simulink model "pendelbeo"  (R2012b)
settings: Solver=ode45  StartTime=0.0  StopTime=10.0  RelTol=1e-3
undefined symbols (not defined in the file): g, J_S0, l, m, M, p, x1, x2, x3, x4
libraries: commnoisgen2 x1
settings Model: Creator=Pendel  LastModifiedBy=Pendel

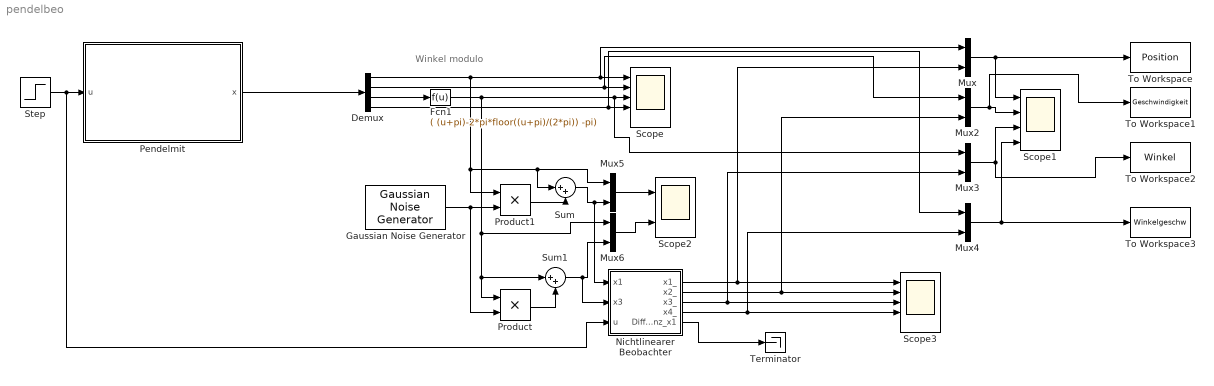
== system pendelbeo ==
  note: Winkel modulo
  Demux : Demux
  Fcn1 : Fcn  Expr=( (u+pi)-2*pi*floor((u+pi)/(2*pi)) -pi)
  Gaussian Noise Generator : commnoisgen2/Gaussian Noise Generator  m=0  d=0.0008  s=0  Ts=1e-3  frameBased=off  sampPerFrame=1  orient=off  outDataType=double
  Mux{,2..6} (6 alike) : Mux  Inputs=2
  Nichtlinearer Beobachter : Subsystem
  Pendelmit : Subsystem
  Product : Product  RndMeth=Zero
  Product1 : Product  RndMeth=Zero
  Scope : Scope  NumInputPorts=5
      settings: TimeRange=100  YMin=-0.5~-2~-5~-20~-200  YMax=1~1~5~40~200  SaveName=simulation_data  MaxDataPoints=500000
  Scope1 : Scope  NumInputPorts=4
      settings: TimeRange=3.23208722741433  YMin=-0.0035~-0.02~-0.0025~-0.0125  YMax=0.003~0.025~0.0025~0.015  SaveName=simulation_data2  MaxDataPoints=500000
  Scope2 : Scope  NumInputPorts=2
      settings: TimeRange=100  YMin=-0.5~-5  YMax=1~5  SaveName=simulation_data4  MaxDataPoints=500000
  Scope3 : Scope  NumInputPorts=5
      settings: TimeRange=25  YMin=-0.5~-2~-4~-200~-1  YMax=0.5~2~4~200~1  SaveName=simulation_data1  MaxDataPoints=500000
  Step : Step  SampleTime=0
  Sum : Sum  Inputs=|++
  Sum1 : Sum  Inputs=|++
  Terminator : Terminator
  To Workspace : ToWorkspace  VariableName=Position  SampleTime=-1  SaveFormat=Timeseries
  To Workspace1 : ToWorkspace  VariableName=Geschwindigkeit  SampleTime=-1  SaveFormat=Timeseries
  To Workspace2 : ToWorkspace  VariableName=Winkel  SampleTime=-1  SaveFormat=Timeseries
  To Workspace3 : ToWorkspace  VariableName=Winkelgeschw  SampleTime=-1  SaveFormat=Timeseries
  wires:
  Demux/1 -> Mux5/1, Sum/1, Product1/1, Mux/1, Scope/1
  Demux/4 -> Mux4/1, Scope/4
  Demux/2 -> Mux2/1, Scope/2
  Demux/3 -> Fcn1/1
  Fcn1/1 -> Mux6/1, Sum1/1, Product/1, Mux3/1, Scope/3
  Pendelmit/1(x) -> Demux/1
  Nichtlinearer Beobachter/1(x1_) -> Mux/2, Scope3/1
  Nichtlinearer Beobachter/2(x2_) -> Mux2/2, Scope3/2
  Nichtlinearer Beobachter/3(x3_) -> Mux3/2, Scope3/3
  Nichtlinearer Beobachter/4(x4_) -> Mux4/2, Scope3/4
  Mux3/1 -> Scope1/3, To Workspace2/1
  Mux/1 -> To Workspace/1, Scope1/1
  Mux4/1 -> To Workspace3/1, Scope1/4
  Mux5/1 -> Scope2/1
  Mux6/1 -> Scope2/2
  Gaussian Noise Generator/1 -> Product1/2, Product/2
  Sum/1 -> Nichtlinearer Beobachter/1(x1), Mux5/2
  Sum1/1 -> Nichtlinearer Beobachter/2(x3), Mux6/2
  Nichtlinearer Beobachter/5(Differenz_x1) -> Terminator/1
  Step/1 -> Nichtlinearer Beobachter/3(u), Pendelmit/1(u)
  Mux2/1 -> To Workspace1/1, Scope1/2
  Product1/1 -> Sum/2
  Product/1 -> Sum1/2

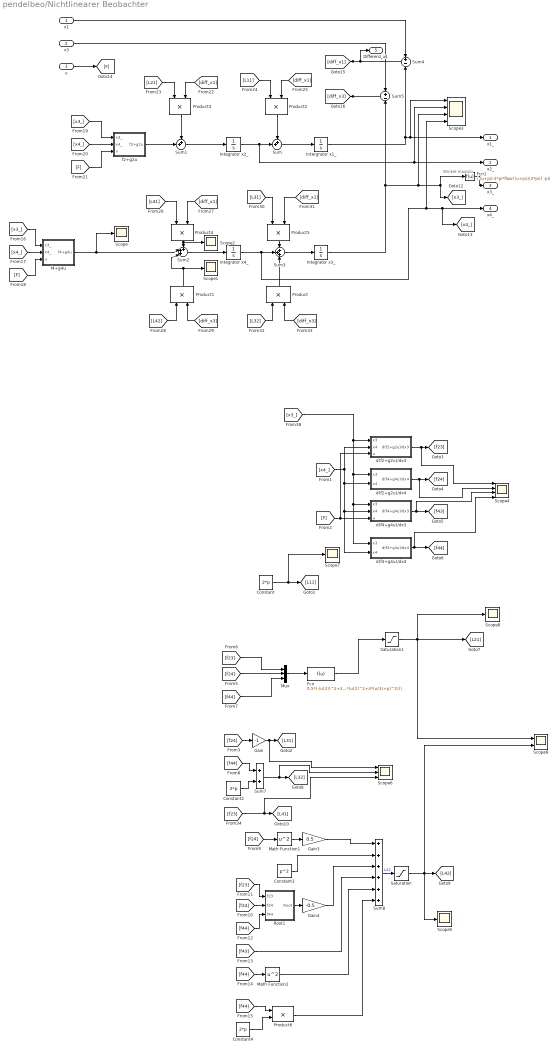
== system pendelbeo/Nichtlinearer Beobachter ==
  note: Winkel modulo
  x1 : Inport
  x3 : Inport  Port=2
  u : Inport  Port=3
  Constant : Constant  Value=2*p
  Constant2 : Constant  Value=2*p
  Constant3 : Constant  Value=p^2
  Constant4 : Constant  Value=2*p
  Fcn : Fcn  Expr=0.5*(-(u(2))^2+2*p^2+sqrt(4*u(1)^2+8*u(1)*u(2)*(u(3)+p)+u(2)^2*(u(2)^2+4*(u(3)+p)^2)))
  Fcn1 : Fcn  Expr=( (u+pi)-2*pi*floor((u+pi)/(2*pi)) -pi)
  Gain : Gain  Gain=-1
  Gain3 : Gain  Gain=0.5
  Gain4 : Gain  Gain=-0.5
  Integrator x2_ : Integrator
  Integrator x3_ : Integrator  InitialCondition=x3
  Integrator x4_ : Integrator
  Intergrator x1_ : Integrator
  Math Function1 : Math  Operator=square  SaturateOnIntegerOverflow=on
  Math Function2 : Math  Operator=square  SaturateOnIntegerOverflow=on
  Mux : Mux  Inputs=3
  Product{,1..6} (7 alike) : Product  SaturateOnIntegerOverflow=on  RndMeth=Zero  InputSameDT=on  OutDataTypeStr=Inherit: Same as first input
  Root1 : Subsystem
  Saturation : Saturate  UpperLimit=5*10^4  LowerLimit=-5*10^4
  Saturation1 : Saturate  UpperLimit=5*10^4  LowerLimit=-5*10^4
  Scope{,1..2,5,7..8} (6 alike) : Scope
      Scope2 settings: SaveName=ScopeData2
      Scope5 settings: SaveName=ScopeData4
      Scope7 settings: SaveName=ScopeData6
      Scope8 settings: SaveName=ScopeData7
  Scope3 : Scope  NumInputPorts=4
      settings: TimeRange=25  YMin=-0.5~-2~-4~-200  YMax=0.5~2~4~200  SaveName=simulation_data3  MaxDataPoints=500000
  Scope4 : Scope  NumInputPorts=4
      settings: YMin=-5~-5~-5~-5  YMax=5~5~5~5  SaveName=ScopeData3
  Scope6 : Scope  NumInputPorts=3
      settings: YMin=-5~-5~-5  YMax=5~5~5  SaveName=ScopeData5
  Scope9 : Scope  NumInputPorts=2
      settings: YMin=-5~-5  YMax=5~5  SaveName=ScopeData8
  Sum : Sum  Inputs=++|  SaturateOnIntegerOverflow=on  InputSameDT=on  OutDataTypeStr=Inherit: Same as first input
  Sum1 : Sum  Inputs=++|  SaturateOnIntegerOverflow=on  InputSameDT=on  OutDataTypeStr=Inherit: Same as first input
  Sum2 : Sum  Inputs=+++|  SaturateOnIntegerOverflow=on  InputSameDT=on  OutDataTypeStr=Inherit: Same as first input
  Sum3 : Sum  Inputs=+++  SaturateOnIntegerOverflow=on  InputSameDT=on  OutDataTypeStr=Inherit: Same as first input
  Sum4 : Sum  Inputs=+-  SaturateOnIntegerOverflow=on  InputSameDT=on  OutDataTypeStr=Inherit: Same as first input
  Sum5 : Sum  Inputs=+-  SaturateOnIntegerOverflow=on  InputSameDT=on  OutDataTypeStr=Inherit: Same as first input
  Sum7 : Sum  SaturateOnIntegerOverflow=on  InputSameDT=on  OutDataTypeStr=Inherit: Same as first input
  Sum8 : Sum  Inputs=++++++  SaturateOnIntegerOverflow=on  InputSameDT=on  OutDataTypeStr=Inherit: Same as first input
  d(f2+g2u)/dx3 : Subsystem
  d(f2+g2u)/dx4 : Subsystem
  d(f4+g4u)/dx3 : Subsystem
  d(f4+g4u)/dx4 : Subsystem
  f2+g2u : Subsystem
  f4+g4u : Subsystem
  x1_ : Outport
  x2_ : Outport  Port=2
  x3_ : Outport  Port=3
  x4_ : Outport  Port=4
  Differenz_x1 : Outport  Port=5
  wires:
  Integrator x2_/1 -> Sum/2, x2_/1, Scope3/2
  Sum/1 -> Intergrator x1_/1
  Sum3/1 -> Integrator x3_/1
  Integrator x4_/1 -> Sum3/2, Scope3/4, [x4_], x4_/1
  Intergrator x1_/1 -> x1_/1, Scope3/1, Sum4/2
  Integrator x3_/1 -> Sum5/2, Scope3/3, [x3_], Fcn1/1
  x1/1 -> Sum4/1
  x3/1 -> Sum5/1
  Product2/1 -> Sum/1
  Product3/1 -> Sum1/1
  Sum2/1 -> Integrator x4_/1
  Sum1/1 -> Integrator x2_/1
  Sum4/1 -> Differenz_x1/1, [diff_x1]
  Sum5/1 -> [diff_x3]
  f2+g2u/1(f2+g2u) -> Sum1/2
  f4+g4u/1(f4+g4u) -> Sum2/2, Scope/1
  u/1 -> [F]
  Product4/1 -> Scope2/1, Sum2/1
  Product5/1 -> Sum3/1
  [L11] -> Product2/1
  [L21] -> Product3/1
  [L31] -> Product5/1
  [L41] -> Product4/1
  [L42] -> Product1/1
  Fcn1/1 -> x3_/1
  [x4_] -> f4+g4u/2(x4_)
  [F] -> f4+g4u/3(u)
  [x4_] -> f2+g2u/2(x4_)
  [F] -> f2+g2u/3(u)
  [diff_x1] -> Product3/2
  [diff_x1] -> Product2/2
  [diff_x1] -> Product4/2
  [diff_x3] -> Product1/2
  [diff_x1] -> Product5/2
  [L32] -> Product/1
  [diff_x3] -> Product/2
  Product/1 -> Sum3/3
  Product1/1 -> Sum2/3, Scope1/1
  [x3_] -> f2+g2u/1(x3_)
  [x3_] -> f4+g4u/1(x3_)
  [x3_] -> d(f4+g4u)/dx4/1(x3), d(f4+g4u)/dx3/1(x3), d(f2+g2u)/dx4/1(x3), d(f2+g2u)/dx3/1(x3)
  [x4_] -> d(f4+g4u)/dx4/2(x4), d(f4+g4u)/dx3/2(x4), d(f2+g2u)/dx4/2(x4), d(f2+g2u)/dx3/2(x4)
  [F] -> d(f2+g2u)/dx3/3(u), d(f4+g4u)/dx3/3(u)
  d(f2+g2u)/dx3/1(d(f2+g2u)/dx3) -> Scope4/1, [f23]
  d(f4+g4u)/dx3/1(d(f4+g4u)/dx3) -> Scope4/3, [f43]
  d(f2+g2u)/dx4/1(d(f4+g4u)/dx4) -> Scope4/2, [f24]
  d(f4+g4u)/dx4/1(d(f4+g4u)/dx4) -> Scope4/4, [f44]
  Constant/1 -> Scope7/1, [L11]
  [f24] -> Gain/1
  Gain/1 -> Scope6/1, [L31]
  [f23] -> Mux/1
  [f24] -> Mux/2
  [f44] -> Mux/3
  Sum7/1 -> Scope6/2, [L32]
  [f44] -> Sum7/1
  Constant2/1 -> Sum7/2
  [f24] -> Math Function1/1
  Math Function1/1 -> Gain3/1
  Gain3/1 -> Sum8/1
  Constant3/1 -> Sum8/2
  Root1/1(Root) -> Gain4/1
  [f23] -> Root1/1(f23)
  [f24] -> Root1/2(f24)
  [f44] -> Root1/3(f44)
  [f44] -> Math Function2/1
  Math Function2/1 -> Sum8/5
  [f44] -> Product6/1
  Constant4/1 -> Product6/2
  Product6/1 -> Sum8/6
  [f23] -> Scope6/3, [L41]
  [f43] -> Sum8/4
  Gain4/1 -> Sum8/3
  Sum8/1 -> Saturation/1  "L42"
  Saturation/1 -> Scope9/2, Scope5/1, [L42]
  Saturation1/1 -> Scope8/1, Scope9/1, [L21]
  Mux/1 -> Fcn/1
  Fcn/1 -> Saturation1/1

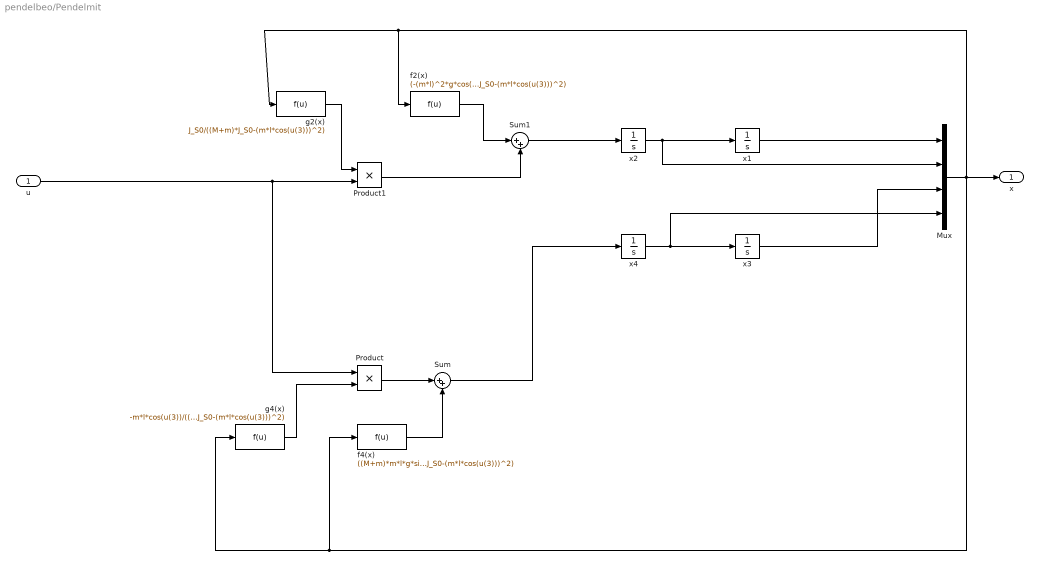
== system pendelbeo/Pendelmit ==
  u : Inport
  Mux : Mux
  Product : Product  RndMeth=Zero
  Product1 : Product  RndMeth=Zero
  Sum : Sum  Inputs=|++
  Sum1 : Sum  Inputs=|++
  f2(x) : Fcn  Expr=(-(m*l)^2*g*cos(u(3))*sin(u(3))+J_S0*m*l*sin(u(3))*u(4)^2)/((M+m)*J_S0-(m*l*cos(u(3)))^2)
  f4(x) : Fcn  Expr=((M+m)*m*l*g*sin(u(3))-(m*l*u(4))^2*cos(u(3))*sin(u(3)))/((M+m)*J_S0-(m*l*cos(u(3)))^2)
  g2(x) : Fcn  Expr=J_S0/((M+m)*J_S0-(m*l*cos(u(3)))^2)
  g4(x) : Fcn  Expr=-m*l*cos(u(3))/((M+m)*J_S0-(m*l*cos(u(3)))^2)
  x1 : Integrator  InitialCondition=x1
  x2 : Integrator  InitialCondition=x2
  x3 : Integrator  InitialCondition=x3
  x4 : Integrator  InitialCondition=x4
  x : Outport
  wires:
  x2/1 -> x1/1, Mux/2
  x4/1 -> Mux/4, x3/1
  x3/1 -> Mux/3
  x1/1 -> Mux/1
  Mux/1 -> x/1, f4(x)/1, g4(x)/1, f2(x)/1, g2(x)/1
  g4(x)/1 -> Product/2
  Product/1 -> Sum/1
  f4(x)/1 -> Sum/2
  Sum/1 -> x4/1
  g2(x)/1 -> Product1/1
  Product1/1 -> Sum1/2
  f2(x)/1 -> Sum1/1
  Sum1/1 -> x2/1
  u/1 -> Product/1, Product1/2

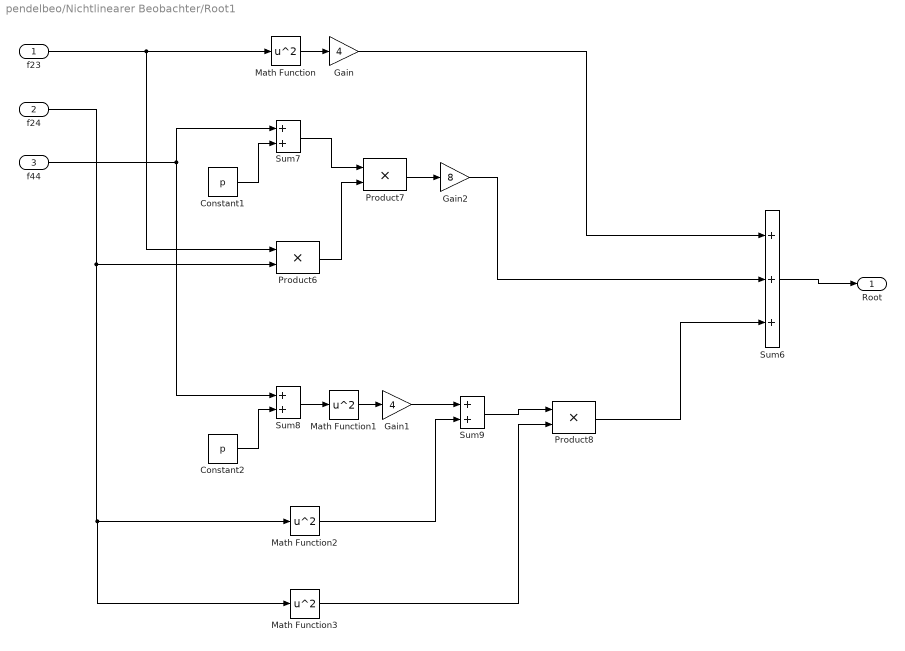
== system pendelbeo/Nichtlinearer Beobachter/Root1 ==
  f23 : Inport
  f24 : Inport  Port=2
  f44 : Inport  Port=3
  Constant1 : Constant  Value=p
  Constant2 : Constant  Value=p
  Gain : Gain  Gain=4
  Gain1 : Gain  Gain=4
  Gain2 : Gain  Gain=8
  Math Function{,1..3} (4 alike) : Math  Operator=square  SaturateOnIntegerOverflow=on
  Product6 : Product  SaturateOnIntegerOverflow=on  RndMeth=Zero  InputSameDT=on  OutDataTypeStr=Inherit: Same as first input
  Product7 : Product  SaturateOnIntegerOverflow=on  RndMeth=Zero  InputSameDT=on  OutDataTypeStr=Inherit: Same as first input
  Product8 : Product  SaturateOnIntegerOverflow=on  RndMeth=Zero  InputSameDT=on  OutDataTypeStr=Inherit: Same as first input
  Sum6 : Sum  Inputs=+++  SaturateOnIntegerOverflow=on  InputSameDT=on  OutDataTypeStr=Inherit: Same as first input
  Sum7 : Sum  SaturateOnIntegerOverflow=on  InputSameDT=on  OutDataTypeStr=Inherit: Same as first input
  Sum8 : Sum  SaturateOnIntegerOverflow=on  InputSameDT=on  OutDataTypeStr=Inherit: Same as first input
  Sum9 : Sum  SaturateOnIntegerOverflow=on  InputSameDT=on  OutDataTypeStr=Inherit: Same as first input
  Root : Outport
  wires:
  Sum8/1 -> Math Function1/1
  Gain1/1 -> Sum9/1
  Sum7/1 -> Product7/1
  Gain/1 -> Sum6/1
  Math Function/1 -> Gain/1
  Math Function1/1 -> Gain1/1
  Sum9/1 -> Product8/1
  Product8/1 -> Sum6/3
  Constant2/1 -> Sum8/2
  f23/1 -> Product6/1, Math Function/1
  Product7/1 -> Gain2/1
  Sum6/1 -> Root/1
  Constant1/1 -> Sum7/2
  Math Function2/1 -> Sum9/2
  Product6/1 -> Product7/2
  Math Function3/1 -> Product8/2
  f24/1 -> Math Function3/1, Math Function2/1, Product6/2
  f44/1 -> Sum8/1, Sum7/1
  Gain2/1 -> Sum6/2

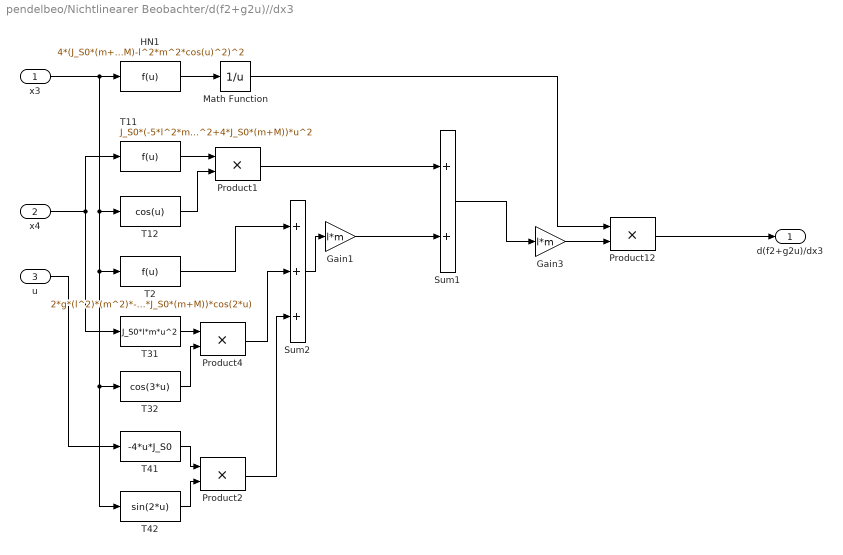
== system pendelbeo/Nichtlinearer Beobachter/d(f2+g2u)//dx3 ==
  x3 : Inport
  x4 : Inport  Port=2
  u : Inport  Port=3
  Gain1 : Gain  Gain=l*m
  Gain3 : Gain  Gain=l*m
  HN1 : Fcn  Expr=4*(J_S0*(m+M)-l^2*m^2*cos(u)^2)^2
  Math Function : Math  Operator=reciprocal  SaturateOnIntegerOverflow=on
  Product{1..2,4,12} (4 alike) : Product  SaturateOnIntegerOverflow=on  RndMeth=Zero  InputSameDT=on  OutDataTypeStr=Inherit: Same as first input
  Sum1 : Sum  SaturateOnIntegerOverflow=on  InputSameDT=on  OutDataTypeStr=Inherit: Same as first input
  Sum2 : Sum  Inputs=+++  SaturateOnIntegerOverflow=on  InputSameDT=on  OutDataTypeStr=Inherit: Same as first input
  T11 : Fcn  Expr=J_S0*(-5*l^2*m^2+4*J_S0*(m+M))*u^2
  T12 : Fcn  Expr=cos(u)
  T2 : Fcn  Expr=2*g*(l^2)*(m^2)*-2*g*(-l^2*m^2+2*J_S0*(m+M))*cos(2*u)
  T31 : Fcn  Expr=J_S0*l*m*u^2
  T32 : Fcn  Expr=cos(3*u)
  T41 : Fcn  Expr=-4*u*J_S0
  T42 : Fcn  Expr=sin(2*u)
  d(f2+g2u)/dx3 : Outport
  wires:
  Math Function/1 -> Product12/1
  HN1/1 -> Math Function/1
  x3/1 -> T42/1, T32/1, T2/1, T12/1, HN1/1
  x4/1 -> T31/1, T11/1
  Product1/1 -> Sum1/1
  T11/1 -> Product1/1
  T12/1 -> Product1/2
  Sum2/1 -> Gain1/1
  T2/1 -> Sum2/1
  T31/1 -> Product4/1
  T32/1 -> Product4/2
  Product4/1 -> Sum2/2
  u/1 -> T41/1
  T41/1 -> Product2/1
  T42/1 -> Product2/2
  Product2/1 -> Sum2/3
  Gain1/1 -> Sum1/2
  Sum1/1 -> Gain3/1
  Product12/1 -> d(f2+g2u)/dx3/1
  Gain3/1 -> Product12/2

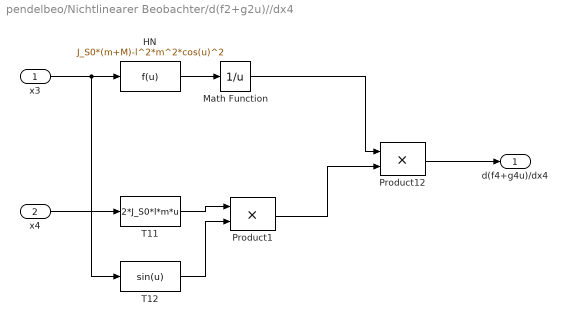
== system pendelbeo/Nichtlinearer Beobachter/d(f2+g2u)//dx4 ==
  x3 : Inport
  x4 : Inport  Port=2
  HN : Fcn  Expr=J_S0*(m+M)-l^2*m^2*cos(u)^2
  Math Function : Math  Operator=reciprocal  SaturateOnIntegerOverflow=on
  Product1 : Product  SaturateOnIntegerOverflow=on  RndMeth=Zero  InputSameDT=on  OutDataTypeStr=Inherit: Same as first input
  Product12 : Product  SaturateOnIntegerOverflow=on  RndMeth=Zero  InputSameDT=on  OutDataTypeStr=Inherit: Same as first input
  T11 : Fcn  Expr=2*J_S0*l*m*u
  T12 : Fcn  Expr=sin(u)
  d(f4+g4u)/dx4 : Outport
  wires:
  Product12/1 -> d(f4+g4u)/dx4/1
  Math Function/1 -> Product12/1
  x4/1 -> T11/1
  HN/1 -> Math Function/1
  x3/1 -> T12/1, HN/1
  T11/1 -> Product1/1
  T12/1 -> Product1/2
  Product1/1 -> Product12/2

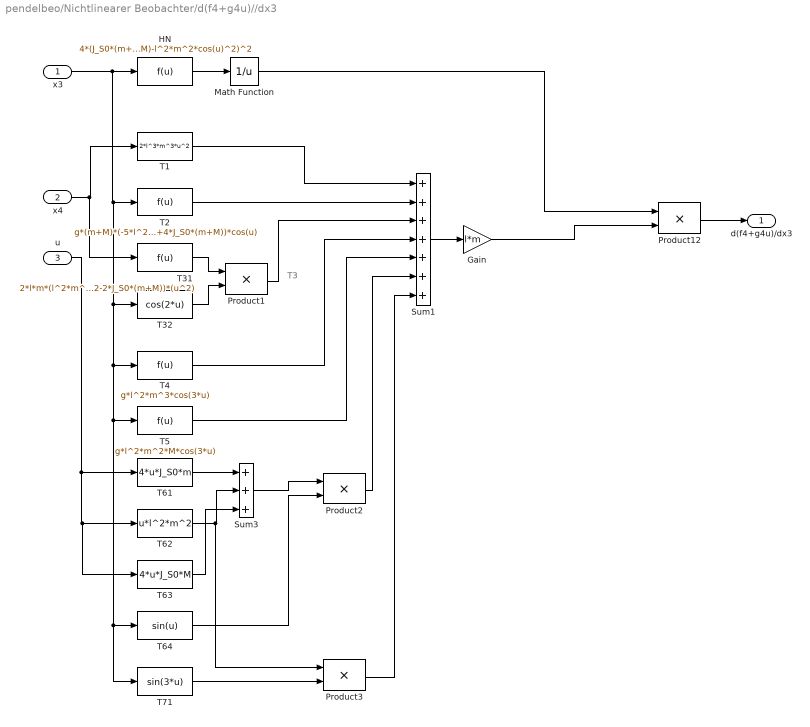
== system pendelbeo/Nichtlinearer Beobachter/d(f4+g4u)//dx3 ==
  note: T3
  x3 : Inport
  x4 : Inport  Port=2
  u : Inport  Port=3
  Gain : Gain  Gain=l*m
  HN : Fcn  Expr=4*(J_S0*(m+M)-l^2*m^2*cos(u)^2)^2
  Math Function : Math  Operator=reciprocal  SaturateOnIntegerOverflow=on
  Product{1..3,12} (4 alike) : Product  SaturateOnIntegerOverflow=on  RndMeth=Zero  InputSameDT=on  OutDataTypeStr=Inherit: Same as first input
  Sum1 : Sum  Inputs=+++++++  SaturateOnIntegerOverflow=on  InputSameDT=on  OutDataTypeStr=Inherit: Same as first input
  Sum3 : Sum  Inputs=+++  SaturateOnIntegerOverflow=on  InputSameDT=on  OutDataTypeStr=Inherit: Same as first input
  T1 : Fcn  Expr=2*l^3*m^3*u^2
  T2 : Fcn  Expr=g*(m+M)*(-5*l^2*m^2+4*J_S0*(m+M))*cos(u)
  T31 : Fcn  Expr=2*l*m*(l^2*m^2-2*J_S0*(m+M))*(u^2)
  T32 : Fcn  Expr=cos(2*u)
  T4 : Fcn  Expr=g*l^2*m^3*cos(3*u)
  T5 : Fcn  Expr=g*l^2*m^2*M*cos(3*u)
  T61 : Fcn  Expr=4*u*J_S0*m
  T62 : Fcn  Expr=u*l^2*m^2
  T63 : Fcn  Expr=4*u*J_S0*M
  T64 : Fcn  Expr=sin(u)
  T71 : Fcn  Expr=sin(3*u)
  d(f4+g4u)/dx3 : Outport
  wires:
  x3/1 -> T71/1, T64/1, T5/1, T4/1, T32/1, T2/1, HN/1
  HN/1 -> Math Function/1
  x4/1 -> T31/1, T1/1
  T31/1 -> Product1/1
  T32/1 -> Product1/2
  T1/1 -> Sum1/1
  T2/1 -> Sum1/2
  Product1/1 -> Sum1/3
  T4/1 -> Sum1/4
  T5/1 -> Sum1/5
  u/1 -> T61/1, T63/1, T62/1
  Product2/1 -> Sum1/6
  T61/1 -> Sum3/1
  T62/1 -> Product3/1, Sum3/2
  T63/1 -> Sum3/3
  Sum3/1 -> Product2/1
  T64/1 -> Product2/2
  T71/1 -> Product3/2
  Product3/1 -> Sum1/7
  Sum1/1 -> Gain/1
  Math Function/1 -> Product12/1
  Gain/1 -> Product12/2
  Product12/1 -> d(f4+g4u)/dx3/1

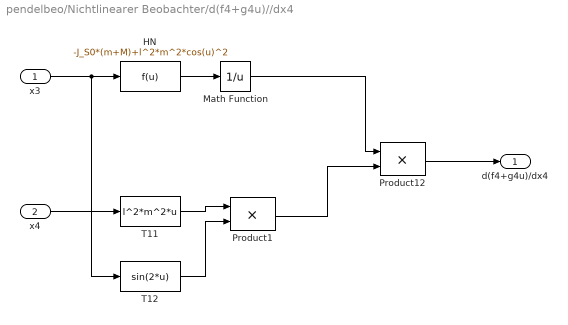
== system pendelbeo/Nichtlinearer Beobachter/d(f4+g4u)//dx4 ==
  x3 : Inport
  x4 : Inport  Port=2
  HN : Fcn  Expr=-J_S0*(m+M)+l^2*m^2*cos(u)^2
  Math Function : Math  Operator=reciprocal  SaturateOnIntegerOverflow=on
  Product1 : Product  SaturateOnIntegerOverflow=on  RndMeth=Zero  InputSameDT=on  OutDataTypeStr=Inherit: Same as first input
  Product12 : Product  SaturateOnIntegerOverflow=on  RndMeth=Zero  InputSameDT=on  OutDataTypeStr=Inherit: Same as first input
  T11 : Fcn  Expr=l^2*m^2*u
  T12 : Fcn  Expr=sin(2*u)
  d(f4+g4u)/dx4 : Outport
  wires:
  Product12/1 -> d(f4+g4u)/dx4/1
  Math Function/1 -> Product12/1
  x4/1 -> T11/1
  HN/1 -> Math Function/1
  x3/1 -> T12/1, HN/1
  T11/1 -> Product1/1
  T12/1 -> Product1/2
  Product1/1 -> Product12/2

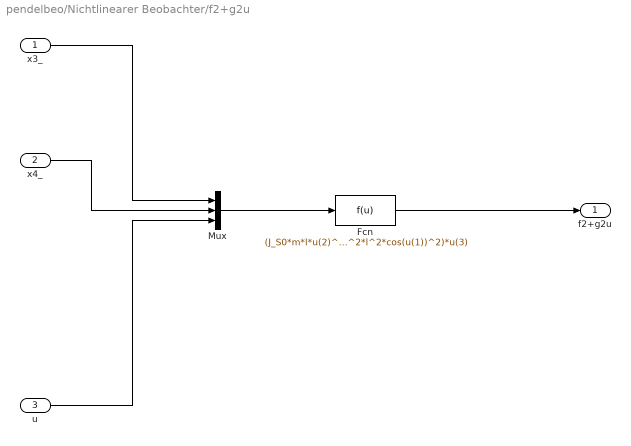
== system pendelbeo/Nichtlinearer Beobachter/f2+g2u ==
  x3_ : Inport
  x4_ : Inport  Port=2
  u : Inport  Port=3
  Fcn : Fcn  Expr=|
      | (J_S0*m*l*u(2)^2*sin(u(1)))/(((M + m)*J_S0 - m^2*l^2 *cos(u(1))^2)) - (m^2*l^2*g*cos(u(1))*sin(u(1)))/((M + m)*J_S0 - m^2*l^2*cos(u(1))^2) + 
      |  J_S0/((M + m)*J_S0 - m^2*l^2*cos(u(1))^2)*u(3)
  Mux : Mux  Inputs=3
  f2+g2u : Outport
  wires:
  Mux/1 -> Fcn/1
  x3_/1 -> Mux/1
  x4_/1 -> Mux/2
  u/1 -> Mux/3
  Fcn/1 -> f2+g2u/1

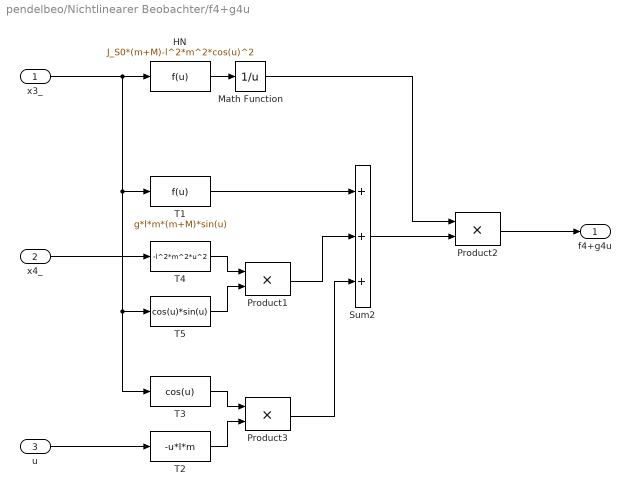
== system pendelbeo/Nichtlinearer Beobachter/f4+g4u ==
  x3_ : Inport
  x4_ : Inport  Port=2
  u : Inport  Port=3
  HN : Fcn  Expr=J_S0*(m+M)-l^2*m^2*cos(u)^2
  Math Function : Math  Operator=reciprocal  SaturateOnIntegerOverflow=on
  Product1 : Product  SaturateOnIntegerOverflow=on  RndMeth=Zero  InputSameDT=on  OutDataTypeStr=Inherit: Same as first input
  Product2 : Product  SaturateOnIntegerOverflow=on  RndMeth=Zero  InputSameDT=on  OutDataTypeStr=Inherit: Same as first input
  Product3 : Product  SaturateOnIntegerOverflow=on  RndMeth=Zero  InputSameDT=on  OutDataTypeStr=Inherit: Same as first input
  Sum2 : Sum  Inputs=+++  SaturateOnIntegerOverflow=on  InputSameDT=on  OutDataTypeStr=Inherit: Same as first input
  T1 : Fcn  Expr=g*l*m*(m+M)*sin(u)
  T2 : Fcn  Expr=-u*l*m
  T3 : Fcn  Expr=cos(u)
  T4 : Fcn  Expr=-l^2*m^2*u^2
  T5 : Fcn  Expr=cos(u)*sin(u)
  f4+g4u : Outport
  wires:
  x3_/1 -> T1/1, T5/1, T3/1, HN/1
  HN/1 -> Math Function/1
  u/1 -> T2/1
  Math Function/1 -> Product2/1
  Sum2/1 -> Product2/2
  Product2/1 -> f4+g4u/1
  T3/1 -> Product3/1
  T2/1 -> Product3/2
  x4_/1 -> T4/1
  T1/1 -> Sum2/1
  T4/1 -> Product1/1
  T5/1 -> Product1/2
  Product1/1 -> Sum2/2
  Product3/1 -> Sum2/3
